simulink model "BEV"  (R2025a)
settings: Solver=FixedStepDiscrete  StartTime=0.0  StopTime=inf  FixedStep=1e-3  RelTol=1e-3
undefined symbols (not defined in the file): DiscIntNeverNeededParam
libraries: simulink x1
settings Model: Creator=mfoua  LastModifiedBy=mfoua

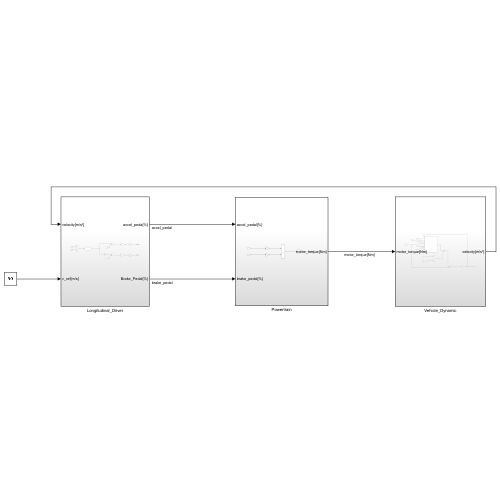
[thumbnail: Simulink's stored preview of the top-level diagram]
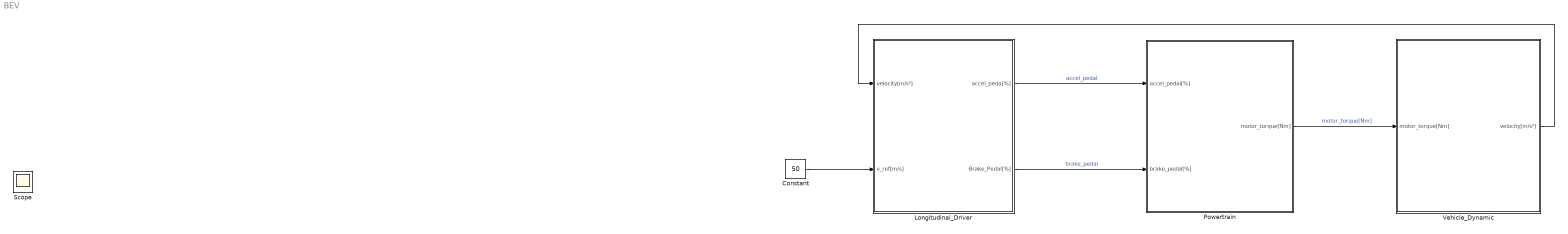
== system BEV ==
  Constant : Constant  Value=50
  Longitudinal_Driver : Subsystem
  Powertrain : Subsystem
  Vehicle_Dynamic : Subsystem
  Scope : Scope
      settings: ActiveDisplayYMinimum=30  ActiveDisplayYMaximum=50
  wires:
  Powertrain/1(motor_torque[Nm]) -> Vehicle_Dynamic/1(motor_torque[Nm])  "motor_torque[Nm]"
  Longitudinal_Driver/1(accel_peda[%]) -> Powertrain/1(accel_pedal[%])  "accel_pedal"
  Longitudinal_Driver/2(Brake_Pedal[%]) -> Powertrain/2(brake_pedal[%])  "brake_pedal"
  Constant/1 -> Longitudinal_Driver/2(v_ref[m/s])
  Vehicle_Dynamic/1(velocity[m/s²]) -> Longitudinal_Driver/1(velocity[m/s²])

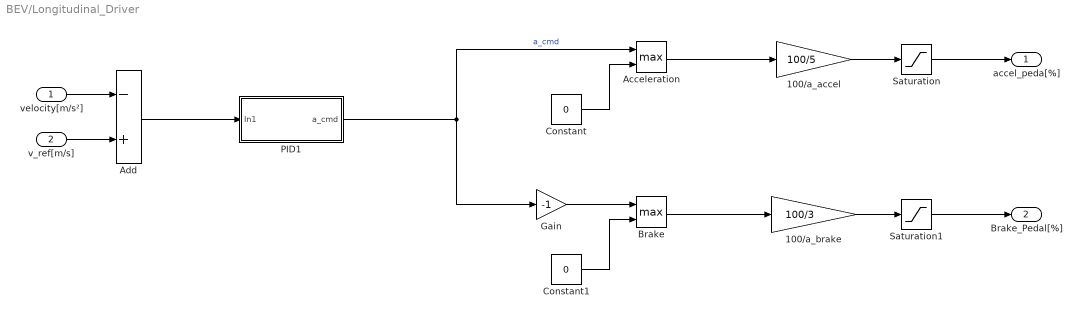
== system BEV/Longitudinal_Driver ==
  velocity[m/s²] : Inport
  v_ref[m/s] : Inport  Port=2
  100/a_accel : Gain  Gain=100/5
  100/a_brake : Gain  Gain=100/3
  Acceleration : MinMax  Function=max  Inputs=2
  Add : Sum  Inputs=-+
  Brake : MinMax  Function=max  Inputs=2
  Constant : Constant  Value=0
  Constant1 : Constant  Value=0
  Gain : Gain  Gain=-1
  PID1 : Subsystem
  Saturation : Saturate  UpperLimit=100  LowerLimit=0
  Saturation1 : Saturate  UpperLimit=100  LowerLimit=0
  accel_peda[%] : Outport
  Brake_Pedal[%] : Outport  Port=2
  wires:
  PID1/1(a_cmd) -> Acceleration/1, Gain/1  "a_cmd"
  Add/1 -> PID1/1(In1)
  100/a_accel/1 -> Saturation/1
  100/a_brake/1 -> Saturation1/1
  Gain/1 -> Brake/1
  Constant/1 -> Acceleration/2
  Constant1/1 -> Brake/2
  Brake/1 -> 100/a_brake/1
  Acceleration/1 -> 100/a_accel/1
  Saturation/1 -> accel_peda[%]/1
  Saturation1/1 -> Brake_Pedal[%]/1
  velocity[m/s²]/1 -> Add/1
  v_ref[m/s]/1 -> Add/2

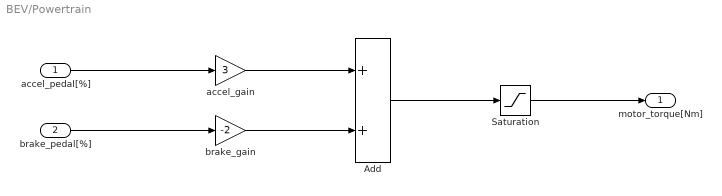
== system BEV/Powertrain ==
  accel_pedal[%] : Inport
  brake_pedal[%] : Inport  Port=2
  Add : Sum
  Saturation : Saturate  UpperLimit=300  LowerLimit=-150
  accel_gain : Gain  Gain=3
  brake_gain : Gain  Gain=-2
  motor_torque[Nm] : Outport
  wires:
  brake_pedal[%]/1 -> brake_gain/1
  accel_pedal[%]/1 -> accel_gain/1
  accel_gain/1 -> Add/1
  brake_gain/1 -> Add/2
  Add/1 -> Saturation/1
  Saturation/1 -> motor_torque[Nm]/1

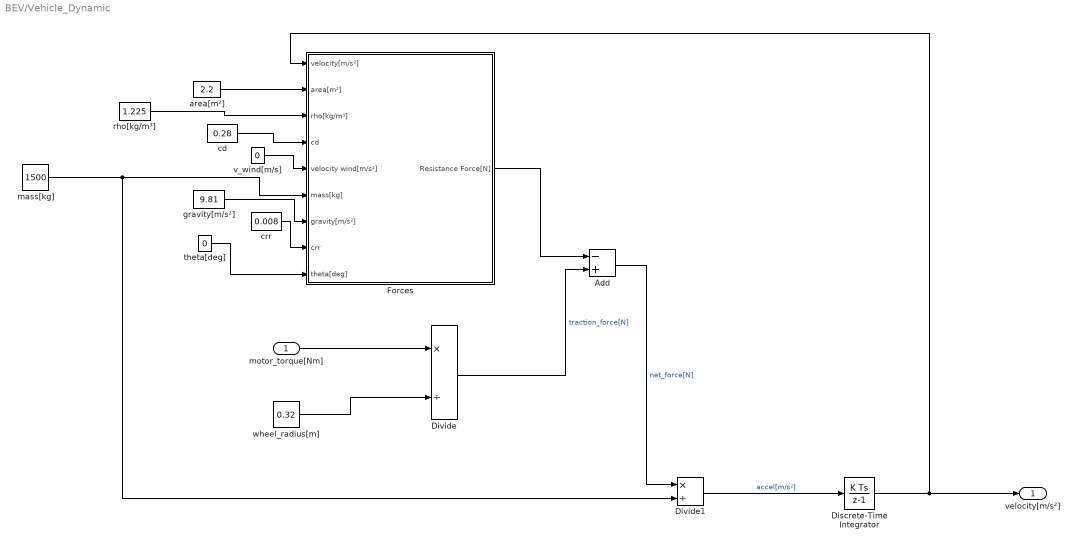
== system BEV/Vehicle_Dynamic ==
  motor_torque[Nm] : Inport
  Add : Sum  Inputs=-+
  Discrete-Time Integrator : DiscreteIntegrator  SampleTime=-1  LimitOutput=on  ICPrevOutput=DiscIntNeverNeededParam  ICPrevScaledInput=DiscIntNeverNeededParam
  Divide : Product  Inputs=*/
  Divide1 : Product  Inputs=*/
  Forces : Subsystem
  area[m²] : Constant  Value=2.2
  cd : Constant  Value=0.28
  crr : Constant  Value=0.008
  gravity[m/s²] : Constant  Value=9.81
  mass[kg] : Constant  Value=1500
  rho[kg/m³] : Constant  Value=1.225
  theta[deg] : Constant  Value=0
  v_wind[m/s] : Constant  Value=0
  wheel_radius[m] : Constant  Value=0.32
  velocity[m/s²] : Outport
  wires:
  motor_torque[Nm]/1 -> Divide/1
  wheel_radius[m]/1 -> Divide/2
  Divide/1 -> Add/2  "traction_force[N]"
  Forces/1(Resistance Force[N]) -> Add/1
  Add/1 -> Divide1/1  "net_force[N]"
  mass[kg]/1 -> Divide1/2, Forces/6(mass[kg])
  Divide1/1 -> Discrete-Time Integrator/1  "accel[m/s²]"
  Discrete-Time Integrator/1 -> Forces/1(velocity[m/s²]), velocity[m/s²]/1
  gravity[m/s²]/1 -> Forces/7(gravity[m/s²])
  area[m²]/1 -> Forces/2(area[m²])
  rho[kg/m³]/1 -> Forces/3(rho[kg/m³])
  cd/1 -> Forces/4(cd)
  v_wind[m/s]/1 -> Forces/5(velocity wind[m/s²])
  crr/1 -> Forces/8(crr)
  theta[deg]/1 -> Forces/9(theta[deg])

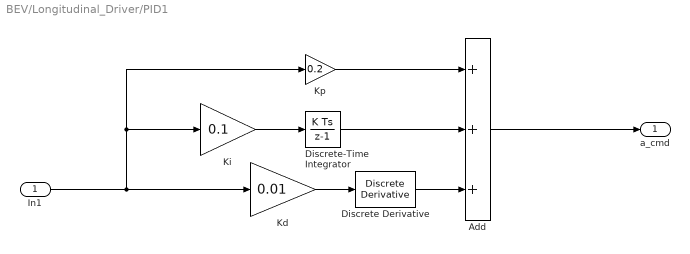
== system BEV/Longitudinal_Driver/PID1 ==
  In1 : Inport
  Add : Sum  Inputs=+++
  Discrete Derivative : simulink/Discrete/Discrete Derivative  gainval=1.0  ICPrevScaledInput=0.0  OutMin=[]  OutMax=[]  OutDataType=fixdt(1, 16)  OutScaling=2^-10  DoSatur=off
  Discrete-Time Integrator : DiscreteIntegrator  SampleTime=-1  ICPrevOutput=DiscIntNeverNeededParam  ICPrevScaledInput=DiscIntNeverNeededParam
  Kd : Gain  Gain=0.01
  Ki : Gain  Gain=0.1
  Kp : Gain  Gain=0.2
  a_cmd : Outport
  wires:
  Discrete Derivative/1 -> Add/3
  Discrete-Time Integrator/1 -> Add/2
  Kd/1 -> Discrete Derivative/1
  Kp/1 -> Add/1
  Ki/1 -> Discrete-Time Integrator/1
  Add/1 -> a_cmd/1
  In1/1 -> Kp/1, Ki/1, Kd/1

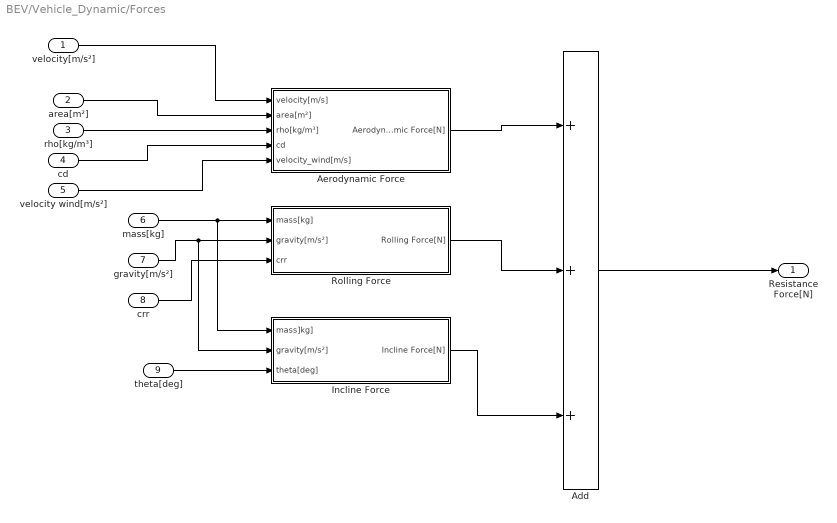
== system BEV/Vehicle_Dynamic/Forces ==
  velocity[m/s²] : Inport
  area[m²] : Inport  Port=2
  rho[kg/m³] : Inport  Port=3
  cd : Inport  Port=4
  velocity wind[m/s²] : Inport  Port=5
  mass[kg] : Inport  Port=6
  gravity[m/s²] : Inport  Port=7
  crr : Inport  Port=8
  theta[deg] : Inport  Port=9
  Add : Sum  Inputs=+++
  Aerodynamic Force : Subsystem
  Incline Force : Subsystem
  Rolling Force : Subsystem
  Resistance Force[N] : Outport
  wires:
  Aerodynamic Force/1(Aerodynamic Force[N]) -> Add/1
  Rolling Force/1(Rolling Force[N]) -> Add/2
  Incline Force/1(Incline Force[N]) -> Add/3
  Add/1 -> Resistance Force[N]/1
  velocity[m/s²]/1 -> Aerodynamic Force/1(velocity[m/s])
  area[m²]/1 -> Aerodynamic Force/2(area[m²])
  rho[kg/m³]/1 -> Aerodynamic Force/3(rho[kg/m³])
  cd/1 -> Aerodynamic Force/4(cd)
  velocity wind[m/s²]/1 -> Aerodynamic Force/5(velocity_wind[m/s])
  mass[kg]/1 -> Incline Force/1(mass]kg]), Rolling Force/1(mass[kg])
  gravity[m/s²]/1 -> Incline Force/2(gravity[m/s²]), Rolling Force/2(gravity[m/s²])
  crr/1 -> Rolling Force/3(crr)
  theta[deg]/1 -> Incline Force/3(theta[deg])

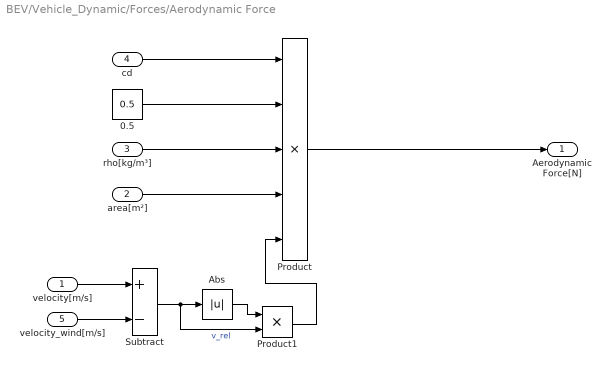
== system BEV/Vehicle_Dynamic/Forces/Aerodynamic Force ==
  velocity[m/s] : Inport
  area[m²] : Inport  Port=2
  rho[kg/m³] : Inport  Port=3
  cd : Inport  Port=4
  velocity_wind[m/s] : Inport  Port=5
  0.5 : Constant  Value=0.5
  Abs : Abs  SaturateOnIntegerOverflow=off
  Product : Product  Inputs=5
  Product1 : Product
  Subtract : Sum  Inputs=+-
  Aerodynamic Force[N] : Outport
  wires:
  0.5/1 -> Product/2
  rho[kg/m³]/1 -> Product/3
  area[m²]/1 -> Product/4
  velocity[m/s]/1 -> Subtract/1
  Product/1 -> Aerodynamic Force[N]/1
  cd/1 -> Product/1
  velocity_wind[m/s]/1 -> Subtract/2
  Subtract/1 -> Product1/2, Abs/1  "v_rel"
  Abs/1 -> Product1/1
  Product1/1 -> Product/5

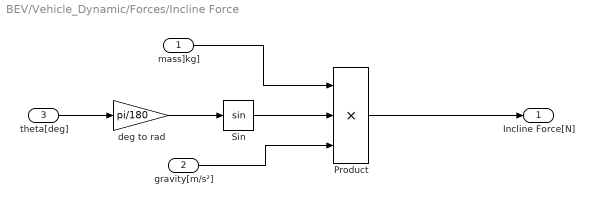
== system BEV/Vehicle_Dynamic/Forces/Incline Force ==
  mass]kg] : Inport
  gravity[m/s²] : Inport  Port=2
  theta[deg] : Inport  Port=3
  Product : Product  Inputs=3
  Sin : Trigonometry
  deg to rad : Gain  Gain=pi/180
  Incline Force[N] : Outport
  wires:
  mass]kg]/1 -> Product/1
  Product/1 -> Incline Force[N]/1
  theta[deg]/1 -> deg to rad/1
  gravity[m/s²]/1 -> Product/3
  Sin/1 -> Product/2
  deg to rad/1 -> Sin/1

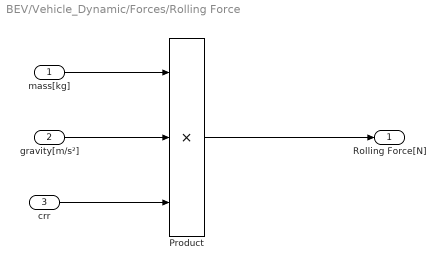
== system BEV/Vehicle_Dynamic/Forces/Rolling Force ==
  mass[kg] : Inport
  gravity[m/s²] : Inport  Port=2
  crr : Inport  Port=3
  Product : Product  Inputs=3
  Rolling Force[N] : Outport
  wires:
  mass[kg]/1 -> Product/1
  gravity[m/s²]/1 -> Product/2
  crr/1 -> Product/3
  Product/1 -> Rolling Force[N]/1
